simulink model "gm_sampleModel1995_3_sub"  (R2023a)
settings: Solver=VariableStepAuto  StartTime=0.0  StopTime=10.0  RelTol=1e-3
libraries: simulink x1, hdlsllib x1
settings Model: Creator=user1  LastModifiedBy=user1
settings OptimizationCC: BlockReduction=off  ConditionallyExecuteInputs=off
settings DebuggingCC: InheritedTsInSrcMsg=none

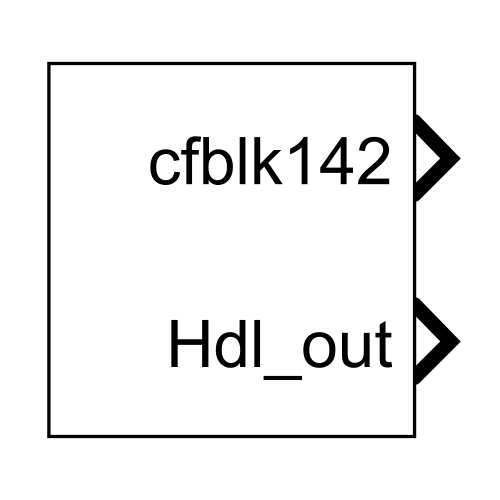
[thumbnail: Simulink's stored preview of the top-level diagram]
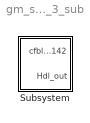
== system gm_sampleModel1995_3_sub ==
  Subsystem : Subsystem

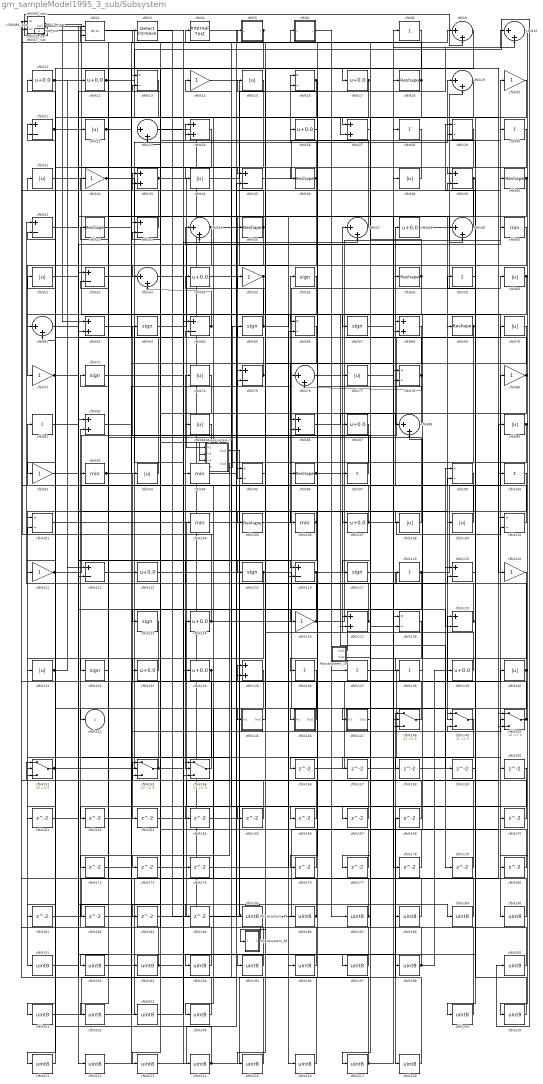
== system gm_sampleModel1995_3_sub/Subsystem ==
  Mysubsystem_16 : Subsystem
  Mysubsystem_39 : Subsystem
  Mysubsystem_49 : Subsystem
  Mysubsystem_7 : Subsystem
  cfblk1 : Constant  Value=0  OutDataTypeStr=uint8  SampleTime=1
  cfblk{9..10,19,23,44,47,49,53,61,76,88} (11 alike) : Sum  Inputs=|++  OutDataTypeStr=uint8
  cfblk{8,28,30,59,81,97,100,118,136..138} (11 alike) : Sum  Inputs=+  OutDataTypeStr=uint8
  cfblk{13,16,29,66,78,95,99,101,110,128} (10 alike) : Product  Inputs=*/  OutDataTypeStr=uint8  RndMeth=Zero  SaturateOnIntegerOverflow=on
  cfblk102_inst : Subsystem
  cfblk{50,92,94,104,106} (5 alike) : MinMax  OutDataTypeStr=uint8
  cfblk{18,36,40,42,45,58,69,96,105} (9 alike) : Reshape
  cfblk{11..12,17,26,48,54,87,107,113,124,133..134,139} (13 alike) : Bias  Bias=0.0  SaturateOnIntegerOverflow=off
  cfblk{15,22,31,34,38,51,60,70,74,77,84,90,93,108..109,131,140} (17 alike) : Abs  OutDataTypeStr=uint8  SaturateOnIntegerOverflow=off
  cfblk{14,20,32,55,71,80,91,111,120,126} (10 alike) : Gain  OutDataTypeStr=uint8
  cfblk{21,35,39,41,43,52,64,75,112,116,119,129} (12 alike) : Sum  Inputs=+-  OutDataTypeStr=uint8
  cfblk{56,63,65,67,72,115,117,123,132} (9 alike) : Signum
  cfblk121_inst : Subsystem
  cfblk{24,27,33,62,68,82,86,127,135} (9 alike) : Sum  OutDataTypeStr=uint8
  cfblk145 : Subsystem
  cfblk146 : Subsystem
  cfblk147 : Subsystem
  cfblk{148..151,153..154} (6 alike) : Switch  OutDataTypeStr=uint8  SaturateOnIntegerOverflow=off  InputSameDT=off
  cfblk{156..168,170,172..174,176..184} (26 alike) : Delay  SampleTime=1
  cfblk{185..198,200..204,209..218} (29 alike) : DataTypeConversion  OutDataTypeStr=uint8  SaturateOnIntegerOverflow=off  RndMeth=Floor
  cfblk2 : RelationalOperator  Operator=<=  OutDataTypeStr=boolean  InputSameDT=off
  cfblk25_inst : Subsystem
  cfblk3 : simulink/Logic and Bit Operations/Detect Increase  vinit=0.0  OutDataTypeStr=uint8
      settings: LibrarySourceBlock=|
      | hdlsllib/Logic and Bit
      | Operations/Detect
      | Increase
  cfblk4 : hdlsllib/Logic and Bit Operations/Interval Test  IntervalClosedRight=on  uplimit=0.5  IntervalClosedLeft=on  lowlimit=-0.5  OutDataTypeStr=uint8
  cfblk5 : Subsystem  mask(Compare To Constant){relop=<=, const=double(3), OutDataTypeStr=uint8, ZeroCross=on}
      mask prompts: relop "Simulink:masks:Operator_MP"; const "Simulink:masks:ConstantValue_MP"; OutDataTypeStr "Simulink:masks:OutputDataType_MP"; ZeroCross "Simulink:masks:EnableZerocrossingDetection_MP"
      mask help: Simulink:masks:CompareToConstant_MD
      mask init:
      | OutDataTypeStr = 'uint8';
      | ZeroCross = 'on';
      | blkName = 'sampleModel1995_3_sub/Subsystem/cfblk5';
      | const = double(3);
      | const_str = '3.0';
      | const_val = double(3);
      | relop = '<=';
      | setValue = 'fixdt(0, 8)';
      | str = '<= 3';
      mask TypeOptions relop: == | ~= | < | <= | >= | >
      mask TypeOptions OutDataTypeStr: Simulink:masks:uint8 | Simulink:masks:boolean
      mask Callback ZeroCross: sl('zeroCrossEnable', gcbh);
      mask Display: disp(str)
  cfblk57_inst : Subsystem
  cfblk6 : Subsystem  mask(Compare To Constant){relop=<=, const=double(3), OutDataTypeStr=uint8, ZeroCross=on}
      mask prompts: relop "Simulink:masks:Operator_MP"; const "Simulink:masks:ConstantValue_MP"; OutDataTypeStr "Simulink:masks:OutputDataType_MP"; ZeroCross "Simulink:masks:EnableZerocrossingDetection_MP"
      mask help: Simulink:masks:CompareToConstant_MD
      mask init:
      | OutDataTypeStr = 'uint8';
      | ZeroCross = 'on';
      | blkName = 'sampleModel1995_3_sub/Subsystem/cfblk6';
      | const = double(3);
      | const_str = '3.0';
      | const_val = double(3);
      | relop = '<=';
      | setValue = 'fixdt(0, 8)';
      | str = '<= 3';
      mask TypeOptions relop: == | ~= | < | <= | >= | >
      mask TypeOptions OutDataTypeStr: Simulink:masks:uint8 | Simulink:masks:boolean
      mask Callback ZeroCross: sl('zeroCrossEnable', gcbh);
      mask Display: disp(str)
  cfblk79_inst : Subsystem
  cfblk83_inst : Subsystem
  cfblk89_inst : Subsystem
  cfblk142 : Outport  OutDataTypeStr=uint8  SampleTime=1  VectorParamsAs1DForOutWhenUnconnected=off
  Hdl_out : Outport  Port=2  OutDataTypeStr=uint8  SampleTime=1
  wires:
  Mysubsystem_16/1(Out1) -> cfblk47/1
  Mysubsystem_16/2(Out2) -> cfblk128/2
  Mysubsystem_39/1(Out1) -> cfblk82/2
  Mysubsystem_49/1(Out1) -> cfblk23/1
  Mysubsystem_7/1(Out1) -> Mysubsystem_49/1(In1)
  Mysubsystem_7/2(Out2) -> cfblk172/1
  cfblk1/1 -> cfblk62/1, cfblk190/1
  cfblk10/1 -> cfblk210/1
  cfblk100/1 -> cfblk191/1
  cfblk101/1 -> cfblk166/1
  cfblk102_inst/1(out1) -> cfblk9/2
  cfblk104/1 -> cfblk189/1
  cfblk105/1 -> cfblk56/1
  cfblk106/1 -> cfblk154/2, cfblk101/1
  cfblk107/1 -> cfblk16/1, cfblk110/2, cfblk81/1
  cfblk108/1 -> cfblk42/1
  cfblk109/1 -> cfblk48/1
  cfblk11/1 -> cfblk149/2, Mysubsystem_7/1(In1)
  cfblk110/1 -> cfblk79_inst/1(in1)
  cfblk111/1 -> cfblk70/1, cfblk99/2
  cfblk112/1 -> cfblk19/1
  cfblk113/1 -> cfblk167/1
  cfblk115/1 -> cfblk149/1, cfblk163/1
  cfblk116/1 -> cfblk68/1, cfblk154/3, cfblk28/1
  cfblk117/1 -> cfblk119/2
  cfblk118/1 -> cfblk80/1, cfblk173/1
  cfblk119/1 -> cfblk197/1
  cfblk12/1 -> cfblk200/1, cfblk110/1
  cfblk120/1 -> cfblk194/1
  cfblk121_inst/1(out1) -> cfblk17/1, cfblk95/2
  cfblk123/1 -> cfblk192/1
  cfblk124/1 -> cfblk79_inst/2(in2), cfblk19/2
  cfblk126/1 -> cfblk74/1, cfblk20/1
  cfblk127/1 -> cfblk77/1, cfblk64/2
  cfblk128/1 -> cfblk217/1
  cfblk129/1 -> cfblk11/1, cfblk55/1
  cfblk13/1 -> cfblk151/3
  cfblk131/1 -> cfblk41/2, cfblk22/1, cfblk112/1
  cfblk132/1 -> cfblk72/1
  cfblk133/1 -> cfblk131/1
  cfblk134/1 -> cfblk151/2, cfblk181/1
  cfblk135/1 -> cfblk211/1
  cfblk136/1 -> cfblk204/1
  cfblk137/1 -> cfblk160/1
  cfblk138/1 -> cfblk118/1
  cfblk139/1 -> cfblk65/1
  cfblk14/1 -> cfblk196/1
  cfblk140/1 -> cfblk41/1, cfblk177/1
  cfblk145/1(Out1) -> cfblk15/1
  cfblk146/1(Out1) -> cfblk83_inst/2(in2)
  cfblk147/1(Out1) -> cfblk97/1
  cfblk148/1 -> cfblk124/1
  cfblk149/1 -> cfblk218/1
  cfblk15/1 -> cfblk91/1
  cfblk150/1 -> cfblk84/1, cfblk52/2, cfblk29/2, cfblk180/1
  cfblk151/1 -> cfblk212/1, cfblk16/2
  cfblk153/1 -> cfblk89_inst/1(in1), cfblk150/2
  cfblk154/1 -> cfblk93/1
  cfblk156/1 -> cfblk129/1
  cfblk157/1 -> cfblk148/1
  cfblk158/1 -> cfblk99/1
  cfblk159/1 -> cfblk39/2
  cfblk16/1 -> cfblk161/1, cfblk146/1(In1)
  cfblk160/1 -> cfblk213/1
  cfblk161/1 -> cfblk62/2
  cfblk162/1 -> cfblk150/1
  cfblk163/1 -> cfblk78/1
  cfblk164/1 -> cfblk119/1
  cfblk165/1 -> cfblk151/1
  cfblk166/1 -> cfblk43/2
  cfblk167/1 -> cfblk83_inst/1(in1)
  cfblk168/1 -> cfblk127/1
  cfblk17/1 -> Mysubsystem_7/2(In2), cfblk106/1
  cfblk170/1 -> cfblk13/2
  cfblk172/1 -> cfblk149/3
  cfblk173/1 -> cfblk150/3
  cfblk174/1 -> cfblk66/2
  cfblk176/1 -> cfblk153/1
  cfblk177/1 -> cfblk153/3
  cfblk178/1 -> cfblk86/2
  cfblk179/1 -> cfblk57_inst/1(in1)
  cfblk18/1 -> cfblk89_inst/2(in2), cfblk107/1
  cfblk180/1 -> cfblk88/2
  cfblk181/1 -> cfblk35/2
  cfblk182/1 -> cfblk68/2
  cfblk183/1 -> cfblk116/2
  cfblk184/1 -> cfblk18/1
  cfblk185/1 -> cfblk90/1
  cfblk186/1 -> Hdl_out/1, cfblk4/1
  cfblk187/1 -> cfblk113/1, cfblk102_inst/1(in1)
  cfblk188/1 -> cfblk6/1(u)
  cfblk189/1 -> cfblk92/1
  cfblk19/1 -> cfblk61/2
  cfblk190/1 -> cfblk104/1
  cfblk191/1 -> cfblk195/1
  cfblk192/1 -> cfblk100/1
  cfblk193/1 -> cfblk47/2, cfblk101/2
  cfblk194/1 -> cfblk25_inst/1(in1)
  cfblk195/1 -> cfblk25_inst/2(in2)
  cfblk196/1 -> cfblk33/1
  cfblk197/1 -> cfblk14/1
  cfblk198/1 -> cfblk52/1, cfblk139/1
  cfblk2/1 -> cfblk120/1
  cfblk20/1 -> cfblk39/1
  cfblk200/1 -> cfblk23/2
  cfblk201/1 -> cfblk45/1
  cfblk202/1 -> cfblk8/1
  cfblk203/1 -> cfblk140/1
  cfblk204/1 -> cfblk82/1
  cfblk209/1 -> cfblk87/1
  cfblk21/1 -> cfblk49/2, cfblk12/1
  cfblk210/1 -> cfblk59/1
  cfblk211/1 -> cfblk31/1
  cfblk212/1 -> cfblk135/1
  cfblk213/1 -> cfblk135/2
  cfblk214/1 -> cfblk21/1, cfblk168/1
  cfblk215/1 -> cfblk24/1
  cfblk216/1 -> cfblk24/2
  cfblk217/1 -> cfblk58/1, cfblk26/1, cfblk121_inst/1(in1)
  cfblk218/1 -> cfblk128/1
  cfblk22/1 -> cfblk27/1, cfblk78/2
  cfblk23/1 -> cfblk198/1
  cfblk24/1 -> cfblk214/1
  cfblk25_inst/1(out1) -> cfblk193/1
  cfblk26/1 -> cfblk176/1
  cfblk27/1 -> cfblk157/1
  cfblk28/1 -> cfblk154/1
  cfblk29/1 -> cfblk53/1
  cfblk3/1 -> cfblk75/1
  cfblk30/1 -> cfblk66/1
  cfblk31/1 -> cfblk186/1
  cfblk32/1 -> cfblk96/1, cfblk216/1, cfblk178/1
  cfblk33/1 -> cfblk44/2, cfblk127/2
  cfblk34/1 -> cfblk10/2
  cfblk35/1 -> cfblk30/1
  cfblk36/1 -> cfblk2/1, Mysubsystem_7/3(In3)
  cfblk38/1 -> cfblk36/1
  cfblk39/1 -> cfblk69/1, cfblk148/3
  cfblk4/1 -> cfblk185/1
  cfblk40/1 -> cfblk148/2, cfblk142/1
  cfblk41/1 -> cfblk13/1
  cfblk42/1 -> cfblk129/2
  cfblk43/1 -> cfblk32/1
  cfblk44/1 -> cfblk95/1, cfblk174/1
  cfblk45/1 -> cfblk121_inst/2(in2), cfblk71/1
  cfblk47/1 -> cfblk102_inst/2(in2)
  cfblk48/1 -> cfblk49/1
  cfblk49/1 -> cfblk29/1
  cfblk5/1(y) -> cfblk183/1, cfblk182/1
  cfblk50/1 -> cfblk145/1(In1)
  cfblk51/1 -> cfblk50/1
  cfblk52/1 -> cfblk9/1
  cfblk53/1 -> cfblk94/1
  cfblk54/1 -> cfblk170/1
  cfblk55/1 -> cfblk202/1, cfblk5/1(u)
  cfblk56/1 -> cfblk111/1
  cfblk57_inst/1(out1) -> cfblk35/1
  cfblk58/1 -> cfblk44/1, cfblk117/1, cfblk3/1
  cfblk59/1 -> cfblk209/1
  cfblk6/1(y) -> cfblk187/1
  cfblk60/1 -> cfblk164/1, cfblk138/1
  cfblk61/1 -> cfblk158/1
  cfblk62/1 -> cfblk116/1
  cfblk63/1 -> cfblk38/1
  cfblk64/1 -> cfblk61/1, cfblk53/2
  cfblk65/1 -> cfblk67/1, cfblk54/1, Mysubsystem_7/4(In4)
  cfblk66/1 -> cfblk105/1
  cfblk67/1 -> cfblk10/1
  cfblk68/1 -> cfblk86/1
  cfblk69/1 -> cfblk153/2, cfblk156/1
  cfblk70/1 -> cfblk147/1(In1)
  cfblk71/1 -> cfblk64/1, cfblk126/1
  cfblk72/1 -> cfblk108/1
  cfblk74/1 -> cfblk134/1
  cfblk75/1 -> cfblk33/2, cfblk21/2
  cfblk76/1 -> cfblk179/1
  cfblk77/1 -> cfblk60/1
  cfblk78/1 -> cfblk76/2, cfblk43/1
  cfblk79_inst/1(out1) -> cfblk27/2
  cfblk8/1 -> cfblk201/1
  cfblk80/1 -> cfblk51/1, cfblk215/1, cfblk123/1
  cfblk81/1 -> cfblk184/1
  cfblk82/1 -> cfblk203/1
  cfblk83_inst/1(out1) -> cfblk34/1, cfblk115/1
  cfblk84/1 -> cfblk133/1
  cfblk86/1 -> cfblk88/1
  cfblk87/1 -> cfblk162/1
  cfblk88/1 -> cfblk57_inst/2(in2)
  cfblk89_inst/1(out1) -> cfblk109/1
  cfblk9/1 -> cfblk165/1
  cfblk90/1 -> cfblk112/2, cfblk137/1
  cfblk91/1 -> cfblk188/1
  cfblk92/1 -> cfblk76/1, cfblk75/2
  cfblk93/1 -> cfblk2/2
  cfblk94/1 -> cfblk40/1
  cfblk95/1 -> Mysubsystem_39/1(In1)
  cfblk96/1 -> cfblk159/1, cfblk136/1
  cfblk97/1 -> cfblk63/1
  cfblk99/1 -> cfblk132/1

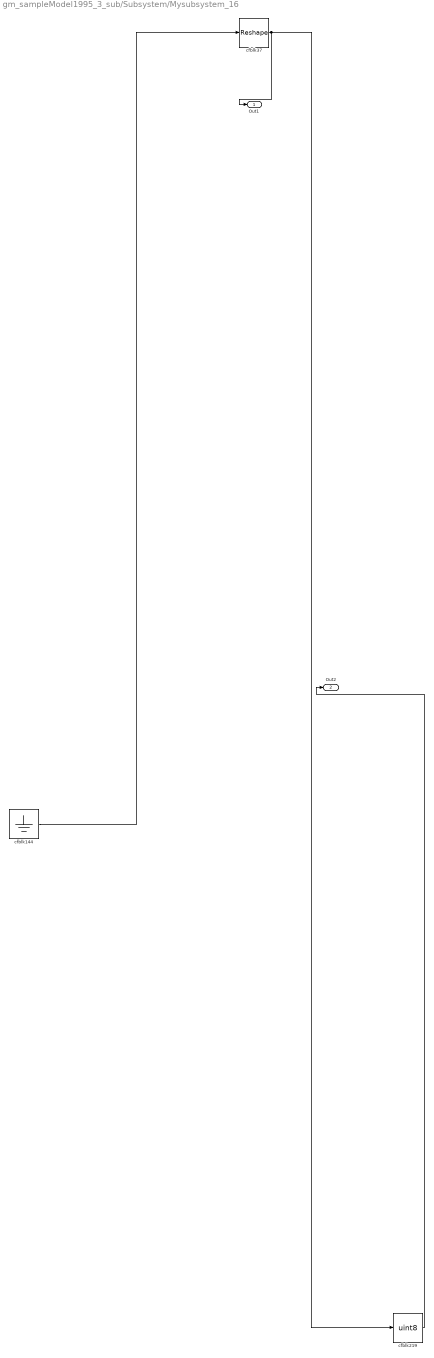
== system gm_sampleModel1995_3_sub/Subsystem/Mysubsystem_16 ==
  cfblk144 : Ground
  cfblk219 : DataTypeConversion  OutDataTypeStr=uint8  SaturateOnIntegerOverflow=off  RndMeth=Floor
  cfblk37 : Reshape
  Out1 : Outport  SampleTime=1
  Out2 : Outport  Port=2  SampleTime=1
  wires:
  cfblk144/1 -> cfblk37/1
  cfblk219/1 -> Out2/1
  cfblk37/1 -> cfblk219/1, Out1/1

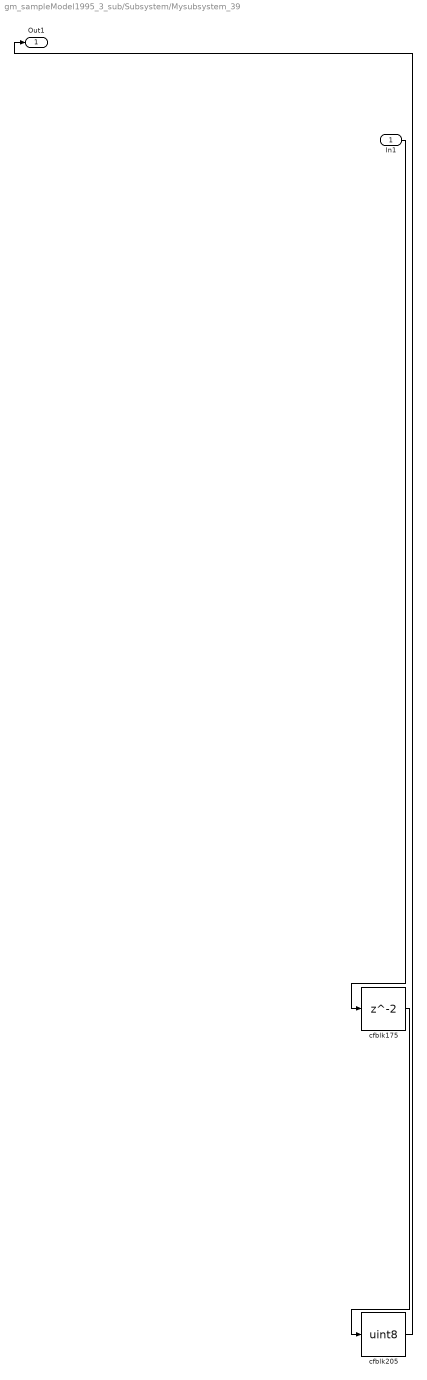
== system gm_sampleModel1995_3_sub/Subsystem/Mysubsystem_39 ==
  In1 : Inport  OutDataTypeStr=uint8  PortDimensions=1  SampleTime=1
  cfblk175 : Delay  SampleTime=1
  cfblk205 : DataTypeConversion  OutDataTypeStr=uint8  SaturateOnIntegerOverflow=off  RndMeth=Floor
  Out1 : Outport  SampleTime=1
  wires:
  In1/1 -> cfblk175/1
  cfblk175/1 -> cfblk205/1
  cfblk205/1 -> Out1/1

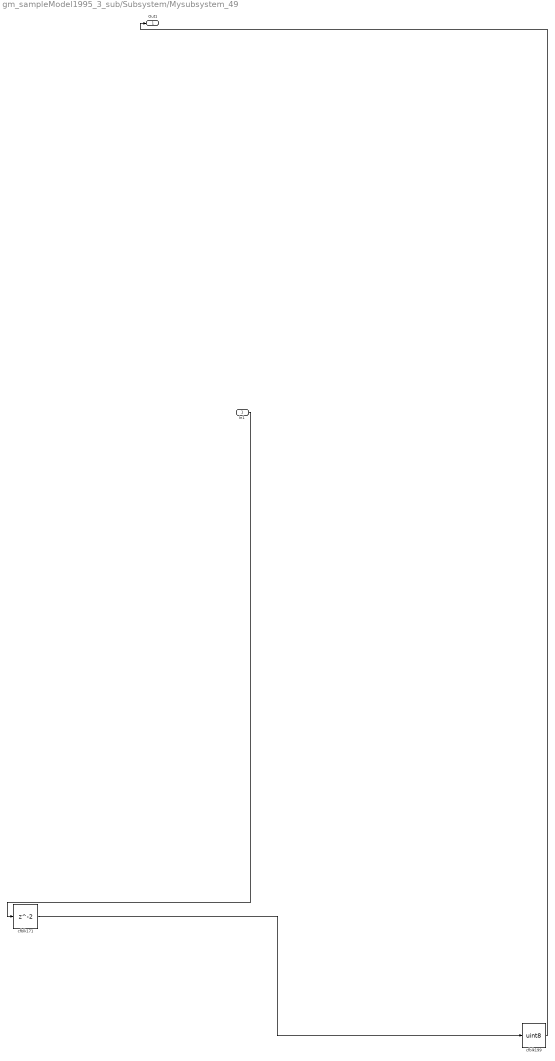
== system gm_sampleModel1995_3_sub/Subsystem/Mysubsystem_49 ==
  In1 : Inport  OutDataTypeStr=uint16  PortDimensions=1  SampleTime=1
  cfblk171 : Delay  SampleTime=1
  cfblk199 : DataTypeConversion  OutDataTypeStr=uint8  SaturateOnIntegerOverflow=off  RndMeth=Floor
  Out1 : Outport  SampleTime=1
  wires:
  In1/1 -> cfblk171/1
  cfblk171/1 -> cfblk199/1
  cfblk199/1 -> Out1/1

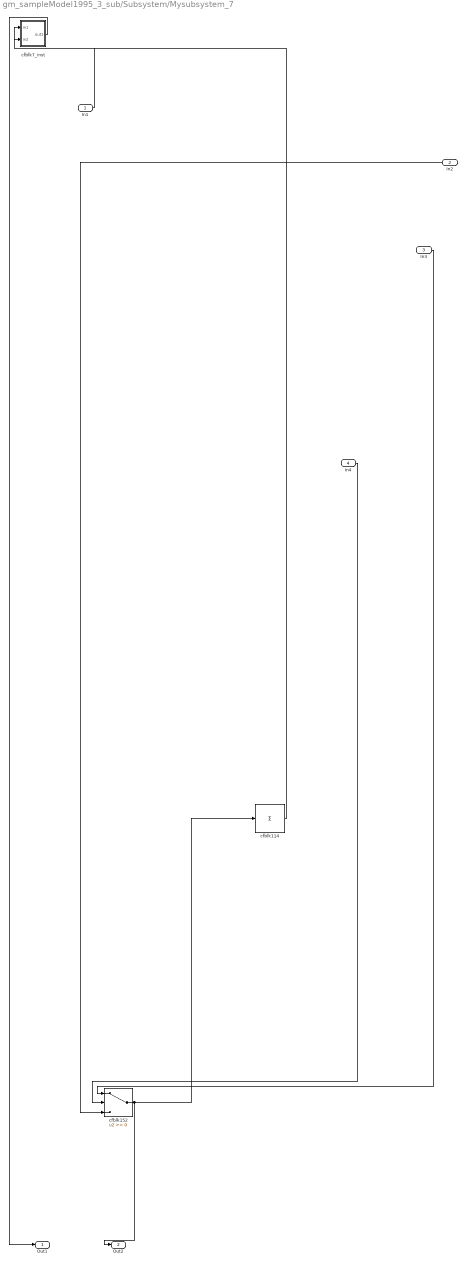
== system gm_sampleModel1995_3_sub/Subsystem/Mysubsystem_7 ==
  In1 : Inport  OutDataTypeStr=uint8  PortDimensions=1  SampleTime=1
  In2 : Inport  Port=2  OutDataTypeStr=uint8  PortDimensions=1  SampleTime=1
  In3 : Inport  Port=3  OutDataTypeStr=uint8  PortDimensions=1  SampleTime=1
  In4 : Inport  Port=4  OutDataTypeStr=uint8  PortDimensions=1  SampleTime=1
  cfblk114 : Sum  Inputs=+
  cfblk152 : Switch  SaturateOnIntegerOverflow=off  InputSameDT=off
  cfblk7_inst : Subsystem
  Out1 : Outport  SampleTime=1
  Out2 : Outport  Port=2  SampleTime=1
  wires:
  In1/1 -> cfblk7_inst/1(in1)
  In2/1 -> cfblk152/3
  In3/1 -> cfblk152/1
  In4/1 -> cfblk152/2
  cfblk114/1 -> cfblk7_inst/2(in2)
  cfblk152/1 -> Out2/1, cfblk114/1
  cfblk7_inst/1(out1) -> Out1/1

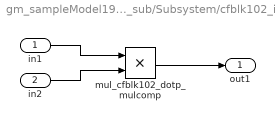
== system gm_sampleModel1995_3_sub/Subsystem/cfblk102_inst ==
  in1 : Inport  OutDataTypeStr=uint8  SampleTime=1
  in2 : Inport  Port=2  OutDataTypeStr=uint8  SampleTime=1
  mul_cfblk102_dotp_mulcomp : Product  Inputs=**  OutDataTypeStr=uint8  SampleTime=1
  out1 : Outport  OutDataTypeStr=uint8  SampleTime=1
  wires:
  in1/1 -> mul_cfblk102_dotp_mulcomp/1
  in2/1 -> mul_cfblk102_dotp_mulcomp/2
  mul_cfblk102_dotp_mulcomp/1 -> out1/1

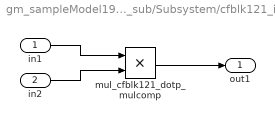
== system gm_sampleModel1995_3_sub/Subsystem/cfblk121_inst ==
  in1 : Inport  OutDataTypeStr=uint8  SampleTime=1
  in2 : Inport  Port=2  OutDataTypeStr=uint8  SampleTime=1
  mul_cfblk121_dotp_mulcomp : Product  Inputs=**  OutDataTypeStr=uint8  SampleTime=1
  out1 : Outport  OutDataTypeStr=uint8  SampleTime=1
  wires:
  in1/1 -> mul_cfblk121_dotp_mulcomp/1
  in2/1 -> mul_cfblk121_dotp_mulcomp/2
  mul_cfblk121_dotp_mulcomp/1 -> out1/1

== system gm_sampleModel1995_3_sub/Subsystem/cfblk145 ==
  In1 : Inport  OutDataTypeStr=uint8  PortDimensions=1  SampleTime=1
  Out1 : Outport  SampleTime=1
  wires:
  In1/1 -> Out1/1

== system gm_sampleModel1995_3_sub/Subsystem/cfblk146 ==
  In1 : Inport  OutDataTypeStr=uint8  PortDimensions=1  SampleTime=1
  Out1 : Outport  SampleTime=1
  wires:
  In1/1 -> Out1/1

== system gm_sampleModel1995_3_sub/Subsystem/cfblk147 ==
  In1 : Inport  OutDataTypeStr=uint8  PortDimensions=1  SampleTime=1
  Out1 : Outport  SampleTime=1
  wires:
  In1/1 -> Out1/1

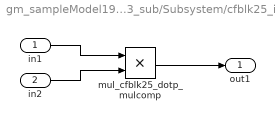
== system gm_sampleModel1995_3_sub/Subsystem/cfblk25_inst ==
  in1 : Inport  OutDataTypeStr=uint8  SampleTime=1
  in2 : Inport  Port=2  OutDataTypeStr=uint8  SampleTime=1
  mul_cfblk25_dotp_mulcomp : Product  Inputs=**  OutDataTypeStr=uint8  SampleTime=1
  out1 : Outport  OutDataTypeStr=uint8  SampleTime=1
  wires:
  in1/1 -> mul_cfblk25_dotp_mulcomp/1
  in2/1 -> mul_cfblk25_dotp_mulcomp/2
  mul_cfblk25_dotp_mulcomp/1 -> out1/1

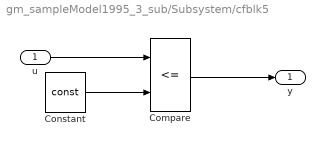
== system gm_sampleModel1995_3_sub/Subsystem/cfblk5 ==
  u : Inport  OutDataTypeStr=uint8  SampleTime=1
  Compare : RelationalOperator  Operator=<=  OutDataTypeStr=fixdt(0, 8)
  Constant : Constant  DisableCoverage=on  Value=const  OutDataTypeStr=Inherit: Inherit via back propagation  SampleTime=-1
  y : Outport  SampleTime=1
  wires:
  u/1 -> Compare/1
  Compare/1 -> y/1
  Constant/1 -> Compare/2

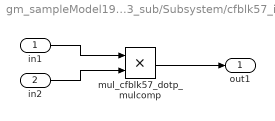
== system gm_sampleModel1995_3_sub/Subsystem/cfblk57_inst ==
  in1 : Inport  OutDataTypeStr=uint8  SampleTime=1
  in2 : Inport  Port=2  OutDataTypeStr=uint8  SampleTime=1
  mul_cfblk57_dotp_mulcomp : Product  Inputs=**  OutDataTypeStr=uint8  SampleTime=1
  out1 : Outport  OutDataTypeStr=uint8  SampleTime=1
  wires:
  in1/1 -> mul_cfblk57_dotp_mulcomp/1
  in2/1 -> mul_cfblk57_dotp_mulcomp/2
  mul_cfblk57_dotp_mulcomp/1 -> out1/1

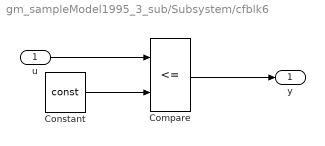
== system gm_sampleModel1995_3_sub/Subsystem/cfblk6 ==
  u : Inport  OutDataTypeStr=uint8  SampleTime=1
  Compare : RelationalOperator  Operator=<=  OutDataTypeStr=fixdt(0, 8)
  Constant : Constant  DisableCoverage=on  Value=const  OutDataTypeStr=Inherit: Inherit via back propagation  SampleTime=-1
  y : Outport  SampleTime=1
  wires:
  u/1 -> Compare/1
  Compare/1 -> y/1
  Constant/1 -> Compare/2

== system gm_sampleModel1995_3_sub/Subsystem/cfblk79_inst ==
  in1 : Inport  OutDataTypeStr=uint8  SampleTime=1
  in2 : Inport  Port=2  OutDataTypeStr=uint8  SampleTime=1
  mul_cfblk79_dotp_mulcomp : Product  Inputs=**  OutDataTypeStr=uint8  SampleTime=1
  out1 : Outport  OutDataTypeStr=uint8  SampleTime=1
  wires:
  in1/1 -> mul_cfblk79_dotp_mulcomp/1
  in2/1 -> mul_cfblk79_dotp_mulcomp/2
  mul_cfblk79_dotp_mulcomp/1 -> out1/1

== system gm_sampleModel1995_3_sub/Subsystem/cfblk83_inst ==
  in1 : Inport  OutDataTypeStr=uint8  SampleTime=1
  in2 : Inport  Port=2  OutDataTypeStr=uint8  SampleTime=1
  mul_cfblk83_dotp_mulcomp : Product  Inputs=**  OutDataTypeStr=uint8  SampleTime=1
  out1 : Outport  OutDataTypeStr=uint8  SampleTime=1
  wires:
  in1/1 -> mul_cfblk83_dotp_mulcomp/1
  in2/1 -> mul_cfblk83_dotp_mulcomp/2
  mul_cfblk83_dotp_mulcomp/1 -> out1/1

== system gm_sampleModel1995_3_sub/Subsystem/cfblk89_inst ==
  in1 : Inport  OutDataTypeStr=uint8  SampleTime=1
  in2 : Inport  Port=2  OutDataTypeStr=uint8  SampleTime=1
  mul_cfblk89_dotp_mulcomp : Product  Inputs=**  OutDataTypeStr=uint8  SampleTime=1
  out1 : Outport  OutDataTypeStr=uint8  SampleTime=1
  wires:
  in1/1 -> mul_cfblk89_dotp_mulcomp/1
  in2/1 -> mul_cfblk89_dotp_mulcomp/2
  mul_cfblk89_dotp_mulcomp/1 -> out1/1

== system gm_sampleModel1995_3_sub/Subsystem/Mysubsystem_7/cfblk7_inst ==
  in1 : Inport  OutDataTypeStr=uint8  SampleTime=1
  in2 : Inport  Port=2  OutDataTypeStr=uint8  SampleTime=1
  mul_cfblk7_dotp_mulcomp : Product  Inputs=**  OutDataTypeStr=uint16  SampleTime=1
  out1 : Outport  OutDataTypeStr=uint16  SampleTime=1
  wires:
  in1/1 -> mul_cfblk7_dotp_mulcomp/1
  in2/1 -> mul_cfblk7_dotp_mulcomp/2
  mul_cfblk7_dotp_mulcomp/1 -> out1/1
